simulink model "weeek2prob4"  (R2020a)
settings: Solver=VariableStepAuto  StartTime=0.0  StopTime=10.0  RelTol=1e-3
PreLoadFcn:
  | Kp=97.1186;
  | Ki=4810.1436;
  | Kd=0.489767;
  | N=119827;
  | b=3.5077E-6;
  | R=4;
  | L=2.75E-6;
  | K=0.0274;
  | J=3.2284E-6
settings Model: DataDictionary=weeekk2prob4.sldd  Creator=Admin  LastModifiedBy=Admin

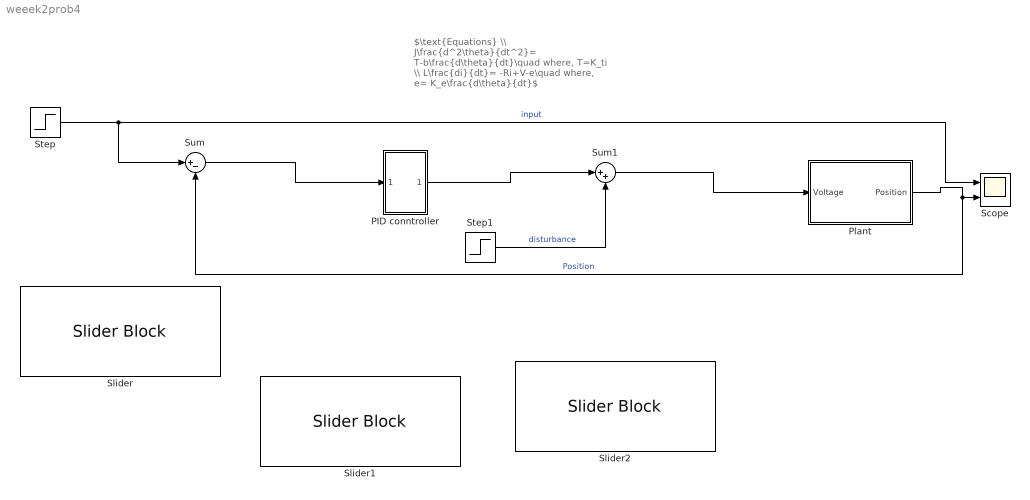
== system weeek2prob4 ==
  note: $\text{Equations} \\ J\frac{d^2\theta}{dt^2}= T-b\frac{d\theta}{dt}\quad where, T=K_ti \\ L\frac{di}{dt}= -Ri+V-e\quad where, e= K_e\frac{d\theta}{dt}$
  PID conntroller : ModelReference  ModelNameDialog=pidcontrolller  SimulationMode=Normal  ModelReferenceVersion=1.6
  Plant : Subsystem
  Scope : Scope  NumInputPorts=2
  Slider : SliderBlock
  Slider1 : SliderBlock
  Slider2 : SliderBlock
  Step : Step  SampleTime=0
  Step1 : Step  SampleTime=0
  Sum : Sum  Inputs=|+-
  Sum1 : Sum  Inputs=|++
  wires:
  Sum/1 -> PID conntroller/1
  PID conntroller/1 -> Sum1/1
  Step1/1 -> Sum1/2  "disturbance"
  Sum1/1 -> Plant/1(Voltage)
  Plant/1(Position) -> Sum/2, Scope/2  "Position"
  Step/1 -> Scope/1, Sum/1  "input"

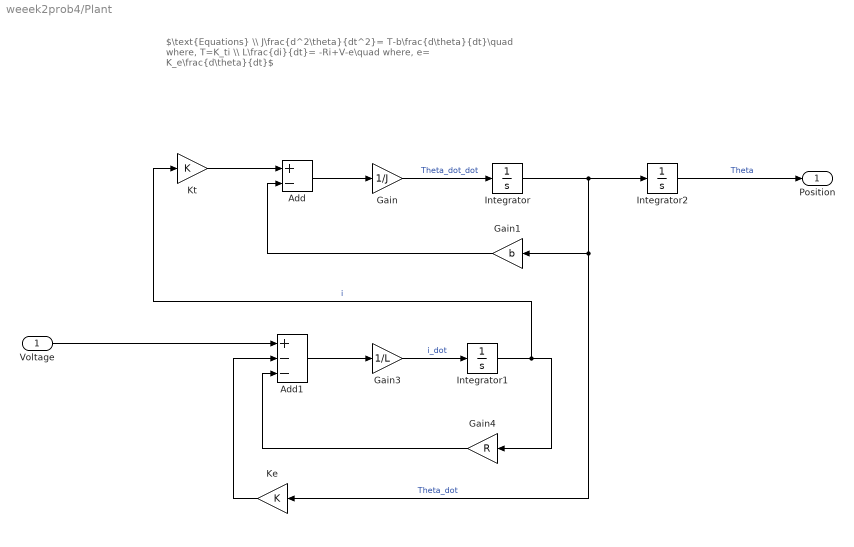
== system weeek2prob4/Plant ==
  note: $\text{Equations} \\ J\frac{d^2\theta}{dt^2}= T-b\frac{d\theta}{dt}\quad where, T=K_ti \\ L\frac{di}{dt}= -Ri+V-e\quad where, e= K_e\frac{d\theta}{dt}$
  Voltage : Inport
  Add : Sum  Inputs=+-
  Add1 : Sum  Inputs=+--
  Gain : Gain  Gain=1/J
  Gain1 : Gain  Gain=b
  Gain3 : Gain  Gain=1/L
  Gain4 : Gain  Gain=R
  Integrator : Integrator
  Integrator1 : Integrator
  Integrator2 : Integrator
  Ke : Gain  Gain=K
  Kt : Gain  Gain=K
  Position : Outport
  wires:
  Integrator/1 -> Integrator2/1, Ke/1, Gain1/1  "Theta_dot"
  Ke/1 -> Add1/2
  Gain1/1 -> Add/2
  Integrator2/1 -> Position/1  "Theta"
  Kt/1 -> Add/1
  Integrator1/1 -> Kt/1, Gain4/1  "i"
  Gain4/1 -> Add1/3
  Gain/1 -> Integrator/1  "Theta_dot_dot"
  Add1/1 -> Gain3/1
  Gain3/1 -> Integrator1/1  "i_dot"
  Add/1 -> Gain/1
  Voltage/1 -> Add1/1
